simulink model "UAV_NL_model"  (R2024b)
settings: Solver=VariableStepAuto  StartTime=0.0  StopTime=10.0  RelTol=1e-3
values from neighbouring files (symbols this model uses):
  g = 9.81    [main.m]    (also in quadrotorStepFunction.m)
  Ixx = 0.01    [main.m]    (also in quadrotorStepFunction.m)
  Iyy = 0.01    [main.m]    (also in quadrotorStepFunction.m)
  Izz = 0.02    [main.m]    (also in quadrotorStepFunction.m)
  Kd = diag([17.480  , 11.554 , 20.4670])    [main.m]
  Kd_ang = diag([50, 50, 30])    [main.m]    (also in quadrotorStepFunction.m = diag([50 50 30]))
  Kp = diag([14.908 ,  9.856  , 18.875])    [main.m]
  Kp_ang = diag([150, 150, 100])    [main.m]    (also in quadrotorStepFunction.m = diag([150 150 100]))
  m = 1.5    [main.m]    (also in quadrotorStepFunction.m = 1)
undefined symbols (not defined in the file or in its folder): Ax, Ay, Az
settings Model: Creator=Feder  LastModifiedBy=Alessandro

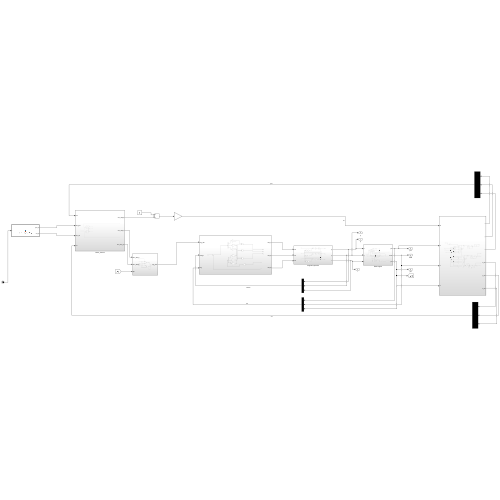
[thumbnail: Simulink's stored preview of the top-level diagram]
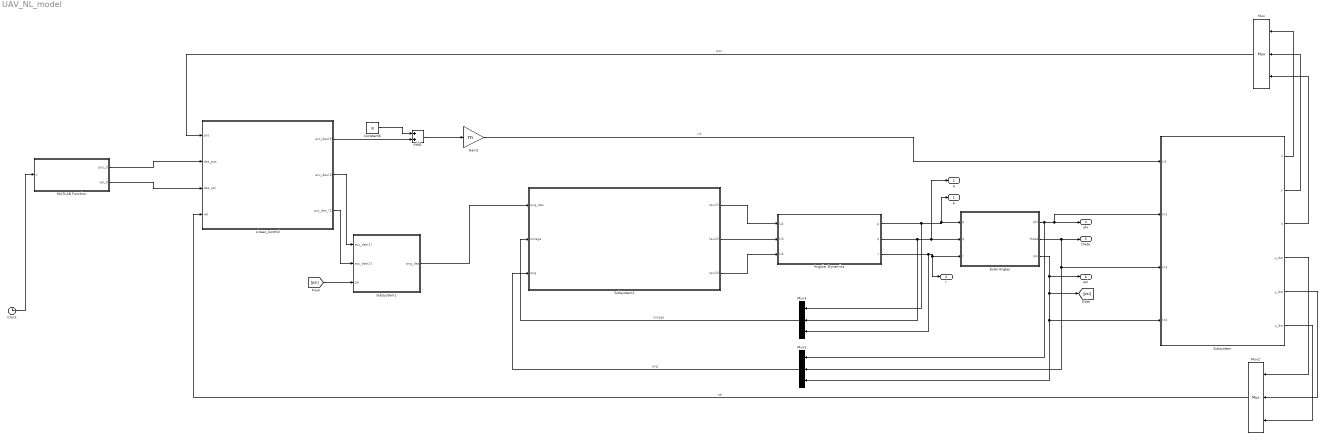
== system UAV_NL_model ==
  Add1 : Sum
  Angular Dynamics : Subsystem
  Clock : Clock
  Constant6 : Constant  Value=g
  Euler Angles : Subsystem
  Gain2 : Gain  Gain=m
  Linear_Control : Subsystem
  MATLAB Function : MATLAB Function  TreatAsAtomicUnit=on
  Mux{,1..3} (4 alike) : Mux  Inputs=3
  Subsystem : Subsystem
  Subsystem1 : Subsystem
  Subsystem2 : Subsystem
  p : Outport
  q : Outport  Port=2
  r : Outport  Port=3
  phi : Outport  Port=4
  theta : Outport  Port=5
  psi : Outport  Port=6
  wires:
  Angular Dynamics/1(p) -> Mux3/1, p/1, Euler Angles/1(p)
  Angular Dynamics/2(q) -> Mux3/2, Euler Angles/2(q), q/1
  Angular Dynamics/3(r) -> Mux3/3, r/1, Euler Angles/3(r)
  Euler Angles/1(phi) -> phi/1, Subsystem/2(In2), Mux1/1
  Euler Angles/2(theta) -> Mux1/2, Subsystem/3(In3), theta/1
  Euler Angles/3(psi) -> [psi], Mux1/3, Subsystem/4(In4), psi/1
  Gain2/1 -> Subsystem/1(U1)  "U1"
  Subsystem/1(x) -> Mux/1
  Subsystem/2(y) -> Mux/2
  Subsystem/3(z) -> Mux/3
  Subsystem/4(x_dot) -> Mux2/1
  Subsystem/5(y_dot) -> Mux2/2
  Subsystem/6(z_dot) -> Mux2/3
  Constant6/1 -> Add1/1
  Add1/1 -> Gain2/1
  Mux/1 -> Linear_Control/1(pos)  "pos"
  Mux2/1 -> Linear_Control/4(vel)  "vel"
  Linear_Control/1(acc_des(3)) -> Add1/2
  Linear_Control/2(acc_des(1)) -> Subsystem1/1(acc_des(1))
  Linear_Control/3(acc_des_(2)) -> Subsystem1/2(acc_des(2))
  [psi] -> Subsystem1/3(psi)
  Subsystem1/1(ang_des) -> Subsystem2/1(ang_des)
  Mux3/1 -> Subsystem2/2(omega)  "omega"
  Mux1/1 -> Subsystem2/3(ang)  "ang"
  Subsystem2/1(tau(1)) -> Angular Dynamics/1(U2)
  Subsystem2/2(tau(2)) -> Angular Dynamics/2(U3)
  Subsystem2/3(tau(3)) -> Angular Dynamics/3(U4)
  Clock/1 -> MATLAB Function/1(t)
  MATLAB Function/1(pos_d) -> Linear_Control/2(des_pos)
  MATLAB Function/2(vel_d) -> Linear_Control/3(des_vel)

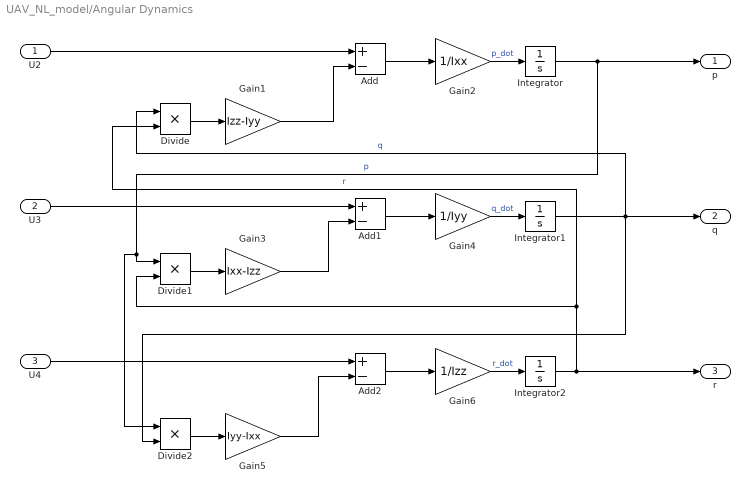
== system UAV_NL_model/Angular Dynamics ==
  U2 : Inport
  U3 : Inport  Port=2
  U4 : Inport  Port=3
  Add : Sum  Inputs=+-
  Add1 : Sum  Inputs=+-
  Add2 : Sum  Inputs=+-
  Divide : Product  Inputs=**
  Divide1 : Product  Inputs=**
  Divide2 : Product  Inputs=**
  Gain1 : Gain  Gain=Izz-Iyy
  Gain2 : Gain  Gain=1/Ixx
  Gain3 : Gain  Gain=Ixx-Izz
  Gain4 : Gain  Gain=1/Iyy
  Gain5 : Gain  Gain=Iyy-Ixx
  Gain6 : Gain  Gain=1/Izz
  Integrator : Integrator
  Integrator1 : Integrator
  Integrator2 : Integrator
  p : Outport
  q : Outport  Port=2
  r : Outport  Port=3
  wires:
  Gain4/1 -> Integrator1/1  "q_dot"
  Gain6/1 -> Integrator2/1  "r_dot"
  Integrator2/1 -> r/1, Divide1/2, Divide/2  "r"
  U2/1 -> Add/1
  Divide2/1 -> Gain5/1
  Integrator/1 -> p/1, Divide1/1, Divide2/1  "p"
  Gain2/1 -> Integrator/1  "p_dot"
  Integrator1/1 -> q/1, Divide2/2, Divide/1  "q"
  Add/1 -> Gain2/1
  Gain1/1 -> Add/2
  Divide/1 -> Gain1/1
  Divide1/1 -> Gain3/1
  Add2/1 -> Gain6/1
  U3/1 -> Add1/1
  Add1/1 -> Gain4/1
  Gain3/1 -> Add1/2
  Gain5/1 -> Add2/2
  U4/1 -> Add2/1

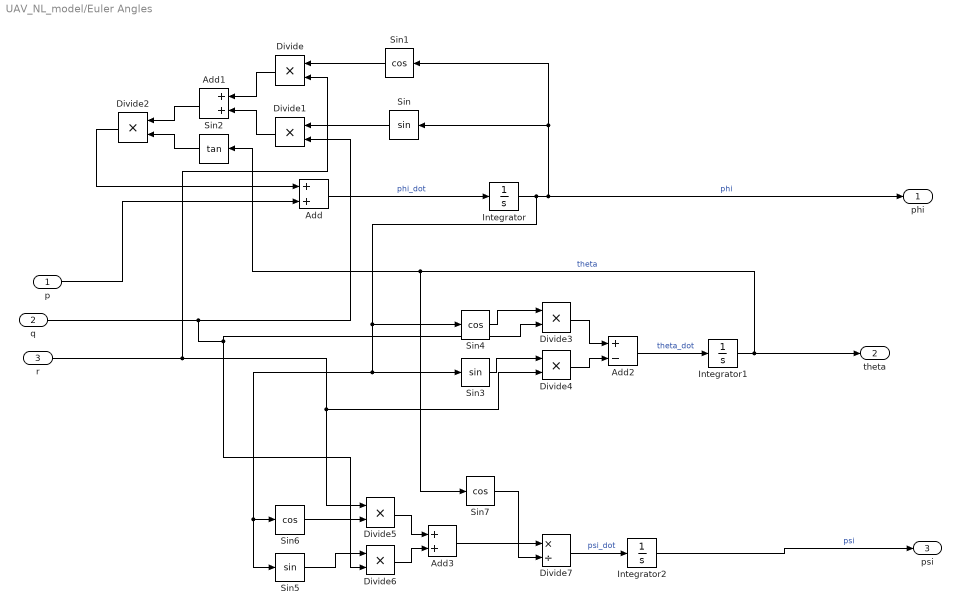
== system UAV_NL_model/Euler Angles ==
  p : Inport
  q : Inport  Port=2
  r : Inport  Port=3
  Add : Sum
  Add1 : Sum
  Add2 : Sum  Inputs=+-
  Add3 : Sum
  Divide{,1..6} (7 alike) : Product  Inputs=**
  Divide7 : Product  Inputs=*/
  Integrator : Integrator
  Integrator1 : Integrator
  Integrator2 : Integrator
  Sin : Trigonometry
  Sin{1,4,6..7} (4 alike) : Trigonometry  Operator=cos
  Sin2 : Trigonometry  Operator=tan
  Sin3 : Trigonometry
  Sin5 : Trigonometry
  phi : Outport
  theta : Outport  Port=2
  psi : Outport  Port=3
  wires:
  Add1/1 -> Divide2/1
  Sin4/1 -> Divide3/1
  Add3/1 -> Divide7/1
  Add/1 -> Integrator/1  "phi_dot"
  Integrator1/1 -> theta/1, Sin7/1, Sin2/1  "theta"
  Sin3/1 -> Divide4/1
  Integrator/1 -> Sin5/1, Sin6/1, Sin3/1, Sin4/1, phi/1, Sin1/1, Sin/1  "phi"
  Add2/1 -> Integrator1/1  "theta_dot"
  Integrator2/1 -> psi/1  "psi"
  Divide6/1 -> Add3/2
  Sin7/1 -> Divide7/2
  r/1 -> Divide5/1, Divide4/2, Divide/2
  p/1 -> Add/2
  Divide/1 -> Add1/1
  Divide7/1 -> Integrator2/1  "psi_dot"
  Sin6/1 -> Divide5/2
  q/1 -> Divide1/2, Divide3/2, Divide6/2
  Divide2/1 -> Add/1
  Divide4/1 -> Add2/2
  Sin/1 -> Divide1/1
  Sin5/1 -> Divide6/1
  Divide3/1 -> Add2/1
  Sin1/1 -> Divide/1
  Divide5/1 -> Add3/1
  Sin2/1 -> Divide2/2
  Divide1/1 -> Add1/2

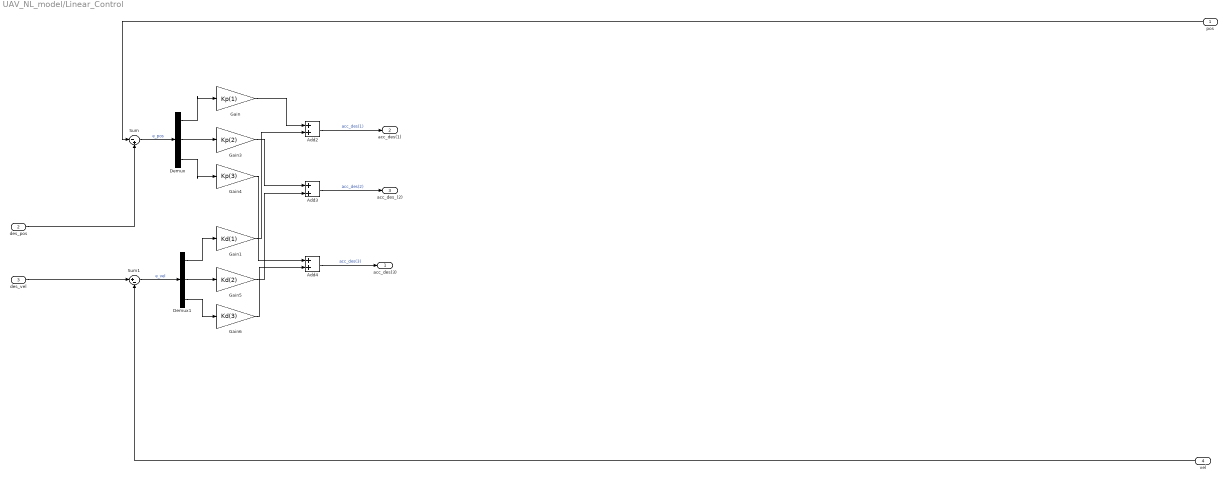
== system UAV_NL_model/Linear_Control ==
  pos : Inport
  des_pos : Inport  Port=2
  des_vel : Inport  Port=3
  vel : Inport  Port=4
  Add2 : Sum
  Add3 : Sum
  Add4 : Sum
  Demux : Demux  Outputs=3
  Demux1 : Demux  Outputs=3
  Gain : Gain  Gain=Kp(1)
  Gain1 : Gain  Gain=Kd(1)
  Gain3 : Gain  Gain=Kp(2)
  Gain4 : Gain  Gain=Kp(3)
  Gain5 : Gain  Gain=Kd(2)
  Gain6 : Gain  Gain=Kd(3)
  Sum : Sum  Inputs=|-+
  Sum1 : Sum  Inputs=|+-
  acc_des(3) : Outport
  acc_des(1) : Outport  Port=2
  acc_des_(2) : Outport  Port=3
  wires:
  Sum/1 -> Demux/1  "e_pos"
  Gain4/1 -> Add4/1
  Sum1/1 -> Demux1/1  "e_vel"
  Add3/1 -> acc_des_(2)/1  "acc_des(2)"
  Gain3/1 -> Add3/1
  Gain6/1 -> Add4/2
  vel/1 -> Sum1/2
  Demux1/2 -> Gain5/1
  Gain/1 -> Add2/1
  Gain1/1 -> Add2/2
  Demux/3 -> Gain4/1
  Demux/2 -> Gain3/1
  Demux1/3 -> Gain6/1
  Demux1/1 -> Gain1/1
  Demux/1 -> Gain/1
  Gain5/1 -> Add3/2
  Add2/1 -> acc_des(1)/1  "acc_des(1)"
  pos/1 -> Sum/1
  des_vel/1 -> Sum1/1
  des_pos/1 -> Sum/2
  Add4/1 -> acc_des(3)/1  "acc_des(3)"

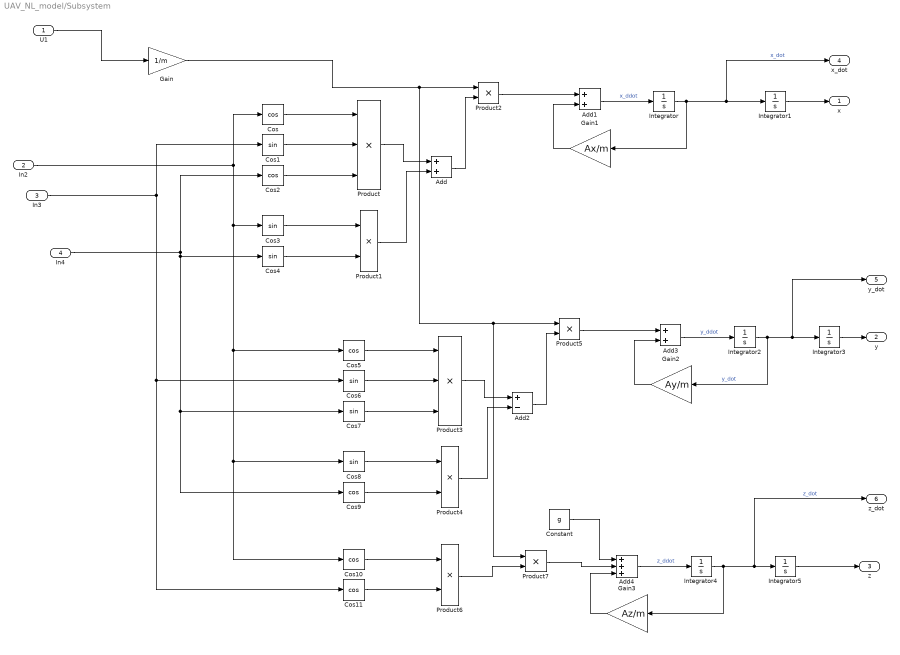
== system UAV_NL_model/Subsystem ==
  U1 : Inport
  In2 : Inport  Port=2
  In3 : Inport  Port=3
  In4 : Inport  Port=4
  Add : Sum
  Add1 : Sum
  Add2 : Sum  Inputs=+-
  Add3 : Sum
  Add4 : Sum  Inputs=+++
  Constant : Constant  Value=g
  Cos{,2,5,9..11} (6 alike) : Trigonometry  Operator=cos
  Cos{1,3..4,6..8} (6 alike) : Trigonometry
  Gain : Gain  Gain=1/m
  Gain1 : Gain  Gain=Ax/m
  Gain2 : Gain  Gain=Ay/m
  Gain3 : Gain  Gain=Az/m
  Integrator{,1..5} (6 alike) : Integrator
  Product : Product  Inputs=3
  Product{1..2,4..7} (6 alike) : Product
  Product3 : Product  Inputs=3
  x : Outport
  y : Outport  Port=2
  z : Outport  Port=3
  x_dot : Outport  Port=4
  y_dot : Outport  Port=5
  z_dot : Outport  Port=6
  wires:
  Cos10/1 -> Product6/1
  In4/1 -> Cos2/1, Cos9/1, Cos7/1, Cos4/1
  Gain1/1 -> Add1/2
  Cos9/1 -> Product4/2
  Add3/1 -> Integrator2/1  "y_ddot"
  In3/1 -> Cos11/1, Cos6/1, Cos1/1
  Integrator/1 -> Gain1/1, x_dot/1, Integrator1/1  "x_dot"
  Product1/1 -> Add/2
  Cos4/1 -> Product1/2
  Cos11/1 -> Product6/2
  Add/1 -> Product2/2
  Product2/1 -> Add1/1
  Product3/1 -> Add2/1
  Cos1/1 -> Product/2
  Product7/1 -> Add4/2
  Product5/1 -> Add3/1
  Product6/1 -> Product7/2
  Cos8/1 -> Product4/1
  Add1/1 -> Integrator/1  "x_ddot"
  Integrator5/1 -> z/1
  Constant/1 -> Add4/1
  Product/1 -> Add/1
  Cos7/1 -> Product3/3
  Product4/1 -> Add2/2
  In2/1 -> Cos/1, Cos10/1, Cos8/1, Cos5/1, Cos3/1
  Gain/1 -> Product7/1, Product5/1, Product2/1
  Gain3/1 -> Add4/3
  Integrator2/1 -> Gain2/1, y_dot/1, Integrator3/1  "y_dot"
  Cos3/1 -> Product1/1
  Integrator1/1 -> x/1
  Cos2/1 -> Product/3
  Add2/1 -> Product5/2
  Cos6/1 -> Product3/2
  Integrator4/1 -> Gain3/1, z_dot/1, Integrator5/1  "z_dot"
  Cos/1 -> Product/1
  U1/1 -> Gain/1
  Add4/1 -> Integrator4/1  "z_ddot"
  Cos5/1 -> Product3/1
  Gain2/1 -> Add3/2
  Integrator3/1 -> y/1

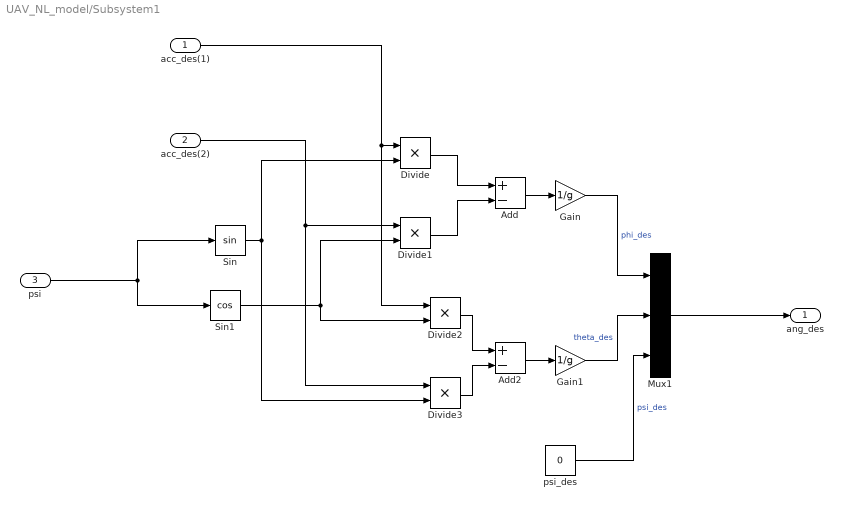
== system UAV_NL_model/Subsystem1 ==
  acc_des(1) : Inport
  acc_des(2) : Inport  Port=2
  psi : Inport  Port=3
  Add : Sum  Inputs=+-
  Add2 : Sum  Inputs=+-
  Divide{,1..3} (4 alike) : Product  Inputs=**
  Gain : Gain  Gain=1/g
  Gain1 : Gain  Gain=1/g
  Mux1 : Mux  Inputs=3
  Sin : Trigonometry
  Sin1 : Trigonometry  Operator=cos
  psi_des : Constant  Value=0
  ang_des : Outport
  wires:
  acc_des(1)/1 -> Divide2/1, Divide/1
  acc_des(2)/1 -> Divide3/1, Divide1/1
  psi/1 -> Sin/1, Sin1/1
  Sin/1 -> Divide/2, Divide3/2
  Divide2/1 -> Add2/1
  Add/1 -> Gain/1
  Sin1/1 -> Divide2/2, Divide1/2
  Divide1/1 -> Add/2
  Divide/1 -> Add/1
  Add2/1 -> Gain1/1
  Divide3/1 -> Add2/2
  Gain/1 -> Mux1/1  "phi_des"
  psi_des/1 -> Mux1/3  "psi_des"
  Gain1/1 -> Mux1/2  "theta_des"
  Mux1/1 -> ang_des/1

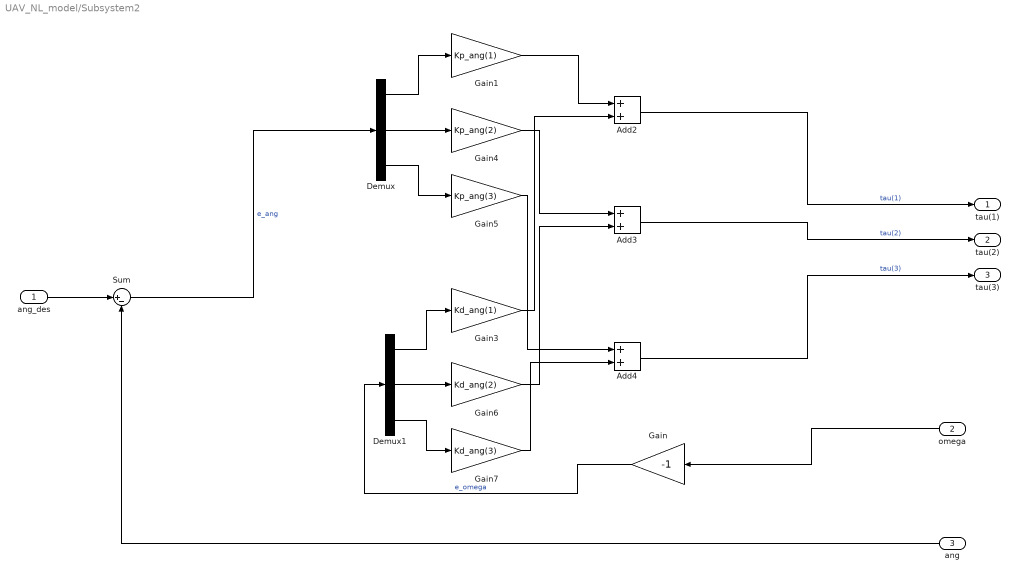
== system UAV_NL_model/Subsystem2 ==
  ang_des : Inport
  omega : Inport  Port=2
  ang : Inport  Port=3
  Add2 : Sum
  Add3 : Sum
  Add4 : Sum
  Demux : Demux  Outputs=3
  Demux1 : Demux  Outputs=3
  Gain : Gain  Gain=-1
  Gain1 : Gain  Gain=Kp_ang(1)
  Gain3 : Gain  Gain=Kd_ang(1)
  Gain4 : Gain  Gain=Kp_ang(2)
  Gain5 : Gain  Gain=Kp_ang(3)
  Gain6 : Gain  Gain=Kd_ang(2)
  Gain7 : Gain  Gain=Kd_ang(3)
  Sum : Sum  Inputs=|+-
  tau(1) : Outport
  tau(2) : Outport  Port=2
  tau(3) : Outport  Port=3
  wires:
  Gain3/1 -> Add2/2
  Demux1/2 -> Gain6/1
  Gain7/1 -> Add4/2
  omega/1 -> Gain/1
  Gain/1 -> Demux1/1  "e_omega"
  Gain4/1 -> Add3/1
  Gain5/1 -> Add4/1
  Demux/1 -> Gain1/1
  Demux/2 -> Gain4/1
  Gain1/1 -> Add2/1
  Demux1/1 -> Gain3/1
  Demux/3 -> Gain5/1
  Demux1/3 -> Gain7/1
  Gain6/1 -> Add3/2
  Sum/1 -> Demux/1  "e_ang"
  ang/1 -> Sum/2
  Add4/1 -> tau(3)/1  "tau(3)"
  Add2/1 -> tau(1)/1  "tau(1)"
  Add3/1 -> tau(2)/1  "tau(2)"
  ang_des/1 -> Sum/1

== matlab function UAV_NL_model/MATLAB Function ==
  data: t input; pos_d output; vel_d output
function [pos_d, vel_d] = reference_trajectory(t)
    % Durata totale della simulazione
    tspan = [0, 15];
    t_ref = linspace(tspan(1), tspan(2), 300);

    % Traiettoria: x = t_ref, y = sin(0.5*t), z = 2 + 0.5*cos(0.5*t)
    ref_traj = [t_ref;
                sin(0.5 * t_ref);
                2 + 0.5 * cos(0.5 * t_ref)];  % 3xN

    % Interpolazione posizione
    pos_d = interp1(t_ref', ref_traj(1:3,:)', t, 'linear', 'extrap')';

    % Derivata numerica per la velocità
    dt = t_ref(2) - t_ref(1);
    vel_traj = gradient(ref_traj(1:3,:), dt);
    vel_d = interp1(t_ref', vel_traj', t, 'linear', 'extrap')';
end
